simulink model "mcb_pmsm_foc_hall_f28069m_Hall_Sensor_Aceleracion"  (R2022b)
settings: Solver=FixedStepDiscrete  StartTime=0.0  StopTime=8  RelTol=1e-3  EnableMultiTasking=on
InitFcn:
  | mcb_pmsm_foc_hall_f28069m_data;
undefined symbols (not defined in the file): Down, GPTRIP1SEL, GPTRIP2SEL, inverter, PI_params, pmsm, target, Ts, Ts_motor, Ts_simulink, Ts_speed, TZ1, TZ2, Up
libraries: simulink x14, mcbcontrolslib x9, mcbpositiondecoderlib x7, idelinklib_common x6, c2802xlib x5, c280xlib x5, slpidlib x3, c2806xlib x3, svdutilitieslib x2, c2000lib x1, mcbplantlib x1, autolibpmsmexterior x1
(part 2 of 3)

== system mcb_pmsm_foc_hall_f28069m_Hall_Sensor_Aceleracion/Hall Sensor C/Capture Event Selection ==
  Hall State : Inport
  If : If  IfExpression=(u1 == 5 | u1 == 6)
  Merge : Merge
  Output 0 : Subsystem  TreatAsAtomicUnit=on
  Output 1 : Subsystem  TreatAsAtomicUnit=on
  Capture Event Select : Outport
  wires:
  Output 1/1(Out1) -> Merge/1
  Output 0/1(Out1) -> Merge/2
  If/2 -> Output 0/Action
  If/1 -> Output 1/Action
  Hall State/1 -> If/1
  Merge/1 -> Capture Event Select/1

== system mcb_pmsm_foc_hall_f28069m_Hall_Sensor_Aceleracion/Hall Sensor C/Code generation ==
  eCAP : c280xlib/eCAP  operatingMode=eCAP  selectCAPx=eCAP3  offsetValue=0  counterSynIn=off  enableCounter=off  syncOutput=Disabled  sampleTime=-1  eventPrescaler=0  selectMode=Continuous  enableOneShot=off  stopValue=Capture Event 2  resetEv1Ts=on  ev1Polarity=Rising Edge  resetEv2Ts=on  ev2Polarity=Falling Edge  resetEv3Ts=off  ev3Polarity=Rising Edge  resetEv4Ts=off  ev4Polarity=Rising Edge  tSCntrDataType=uint32  capEvFlag=off  capFlagDataType=uint16  overFlowFlag=off  overFlowFlagDataType=uint16  periodUnit=Seconds  periodSource=Specify via dialog  waveformPeriod=0.001  dutyUnit=Percentages  dutySource=Specify via dialog  dutyCycle=50  outputPolarity=Active High  enableCEVT1Int=on  enableCEVT2Int=on  enableCEVT3Int=off  enableCEVT4Int=off  enableCTROVFInt=on  enablePRDInt=off  enableCMPInt=off
  eCAP_Out : Outport
  wires:
  eCAP/1 -> eCAP_Out/1

== system mcb_pmsm_foc_hall_f28069m_Hall_Sensor_Aceleracion/Hall Sensor C/CodeGen ==
  Bitwise AND : simulink/Logic and Bit Operations/Bitwise Operator  logicop=AND  UseBitMask=on  BitMask=hex2dec('07000000')  BitMaskRealWorld=Stored Integer
  Data Type Conversion : DataTypeConversion  OutDataTypeStr=uint32  ConvertRealWorld=Stored Integer (SI)  SaturateOnIntegerOverflow=off  RndMeth=Floor
  Memory Copy : idelinklib_common/Memory Copy  copyFrom=Specified source code symbol  copyFromAddressSource=Specify via dialog  copyFromAddress=hex2dec('00001000')  copyFromSrcCode=&GpioDataRegs.GPADAT.all  dataTypeFrom=uint32  dataDimensionFrom=1  useOffsetFrom=off  offsetFromSrc=Specify via dialog  offsetFrom=0  strideFrom=1  copyTo=Output port  copyToAddressSource=Specify via dialog  copyToAddress=hex2dec('00002000')  copyToSrcCode=myVariableDst  dataTypeTo=uint32  useOffsetTo=off  offsetToSrc=Specify via dialog  offsetTo=0  strideTo=1  sampleTime=-1  useInitValue=off  initValueSrc=Specify constant value  initValue=1  initValueSrcCode=myInitValueVariable  useAsMask=off  maskOperator=bitwise AND  useTermValue=off  termValue=1  isRealtimeEnabled=off  emitCCBeforeWrite=off  CCBeforeWrite=/* Custom Code Before Write*/  emitCCAfterWrite=off  CCAfterWrite=/* Custom Code After Write*/
  Shift Arithmetic : ArithShift  BitShiftNumber=24
  Out1 : Outport
  wires:
  Data Type Conversion/1 -> Out1/1
  Shift Arithmetic/1 -> Data Type Conversion/1
  Bitwise AND/1 -> Shift Arithmetic/1
  Memory Copy/1 -> Bitwise AND/1

== system mcb_pmsm_foc_hall_f28069m_Hall_Sensor_Aceleracion/Hall Sensor C/Sim ==
  Data Type Conversion : DataTypeConversion  OutDataTypeStr=uint32  ConvertRealWorld=Stored Integer (SI)  SaturateOnIntegerOverflow=off  RndMeth=Floor
  Ground : Ground
  Out1 : Outport
  wires:
  Data Type Conversion/1 -> Out1/1
  Ground/1 -> Data Type Conversion/1

== system mcb_pmsm_foc_hall_f28069m_Hall_Sensor_Aceleracion/Hall Sensor C/Simulation ==
  Ground : Ground
  Ground1 : Ground
  Mux : Mux  Inputs=2
  Out1 : Outport
  wires:
  Ground1/1 -> Mux/2
  Mux/1 -> Out1/1
  Ground/1 -> Mux/1

== system mcb_pmsm_foc_hall_f28069m_Hall_Sensor_Aceleracion/Hardware Init/Code Generation ==
  Input : Inport
  ADC Calib Enable : Constant  Value=inverter.ADCOffsetCalibEnable
  "Calculate ADC Offset " : Subsystem  Priority=1001  TreatAsAtomicUnit=on
  DRV Enable : Subsystem  Priority=1
  Default ADC Offset : Subsystem  Priority=1001  TreatAsAtomicUnit=on
  NOT : Logic  Operator=NOT  IconShape=distinctive  AllPortsSameDT=off  OutDataTypeStr=boolean
  wires:
  Input/1 -> DRV Enable/1(Input)
  ADC Calib Enable/1 -> "Calculate ADC Offset "/Enable, NOT/1
  NOT/1 -> Default ADC Offset/Enable

== system mcb_pmsm_foc_hall_f28069m_Hall_Sensor_Aceleracion/Hardware Init/Simulation ==
  Input : Inport
  Terminator : Terminator
  wires:
  Input/1 -> Terminator/1

== system mcb_pmsm_foc_hall_f28069m_Hall_Sensor_Aceleracion/Heartbeat LED/Code generation ==
  note: Heartbeat LED 1HZ
  In1 : Inport
  Digital Output1 : c2806xlib/Digital Output  GPIO_Number=GPIO24~GPIO31  GPIO_Bit0=off  GPIO_BIT0_Toggle=off  GPIO_Bit1=off  GPIO_BIT1_Toggle=off  GPIO_Bit2=off  GPIO_BIT2_Toggle=off  GPIO_Bit3=off  GPIO_BIT3_Toggle=off  GPIO_Bit4=off  GPIO_BIT4_Toggle=off  GPIO_Bit5=off  GPIO_BIT5_Toggle=off  GPIO_Bit6=off  GPIO_BIT6_Toggle=off  GPIO_Bit7=on  GPIO_BIT7_Toggle=on
  wires:
  In1/1 -> Digital Output1/1

== system mcb_pmsm_foc_hall_f28069m_Hall_Sensor_Aceleracion/Heartbeat LED/Simulation ==
  In1 : Inport
  Simulation_Terminator : Terminator
  wires:
  In1/1 -> Simulation_Terminator/1

== system mcb_pmsm_foc_hall_f28069m_Hall_Sensor_Aceleracion/Inverter and Motor - Plant Model/Codegeneration ==
  Duty_Cycles : Inport
  Ground : Ground
  Ground1 : Ground
  Terminator : Terminator
  Iab_fb_Sim : Outport  VectorParamsAs1DForOutWhenUnconnected=off
  Pos_fb_Sim : Outport  Port=2  VectorParamsAs1DForOutWhenUnconnected=off
  wires:
  Duty_Cycles/1 -> Terminator/1
  Ground/1 -> Iab_fb_Sim/1
  Ground1/1 -> Pos_fb_Sim/1

== system mcb_pmsm_foc_hall_f28069m_Hall_Sensor_Aceleracion/Inverter and Motor - Plant Model/Simulation ==
  Duty_Cycles : Inport
  Inverter : Subsystem
  Load_Profile (Torque) : Subsystem
  RT1 : RateTransition  Deterministic=off  OutPortSampleTime=Ts_simulink
  RT3 : RateTransition  Deterministic=off  OutPortSampleTime=Ts_simulink
  Rate Transition : RateTransition  Deterministic=off  OutPortSampleTime=Ts_motor
  Rate Transition1 : RateTransition  Deterministic=off  OutPortSampleTime=Ts_motor
  Sensor_Measurements : Subsystem
  Surface Mount PMSM : autolibpmsmexterior/Surface Mount PMSM  port_config=Torque  sim_type=Discrete  Ts=Ts_motor  P=pmsm.p  Rs=pmsm.Rs + inverter.R_board  Ldq_=pmsm.Ld  KConstText=Permanent flux linkage constant (lambda_pm):  lambda_pm=pmsm.FluxPM  Ke=159.9771  Kt=1.323  mechanical=[pmsm.J, pmsm.B, 0]  idq0=[0 0]  theta_init=0  omega_init=0  KConst=pmsm.FluxPM  lambda_pm_calc=pmsm.FluxPM  RefBlkName='autolibpmsmexterior/Surface Mount PMSM'  aMode=5  Ldq="[0.0006      0.0006]"
  Terminator : Terminator
  Iab_fb_Sim : Outport  VectorParamsAs1DForOutWhenUnconnected=off
  Pos_fb_Sim : Outport  Port=2  VectorParamsAs1DForOutWhenUnconnected=off
  wires:
  RT1/1 -> Sensor_Measurements/2(PhaseCurr)
  Surface Mount PMSM/3 -> Terminator/1
  Inverter/1(Vabc) -> Rate Transition/1
  Load_Profile (Torque)/1(Load_Trq) -> Rate Transition1/1
  Surface Mount PMSM/2 -> RT1/1  "Iabc"
  RT3/1 -> Sensor_Measurements/1(Info)
  Surface Mount PMSM/1 -> RT3/1
  Rate Transition1/1 -> Surface Mount PMSM/1
  Rate Transition/1 -> Surface Mount PMSM/2
  Duty_Cycles/1 -> Inverter/1(Duty_abc)
  Sensor_Measurements/1(Iab_fb) -> Iab_fb_Sim/1
  Sensor_Measurements/2(Pos_fb) -> Pos_fb_Sim/1

== system mcb_pmsm_foc_hall_f28069m_Hall_Sensor_Aceleracion/Serial Receive/Code Generation ==
  SCI Receive : c280xlib/SCI Receive  sciModule=A  dataHead=''  headerCheckMaxCount=16  dataTail=''  dataType=uint16  dataLenOptions=Length via dialog  dataDim=2  maxDataLength=1  initValue=0  errOption=Output the last received value  errValue=0  sampleTime=-1  blockingMode=on  timeOut=0.019444  outputStatus=off
  Data : Outport
  wires:
  SCI Receive/1 -> Data/1

== system mcb_pmsm_foc_hall_f28069m_Hall_Sensor_Aceleracion/Serial Receive/Data_Conditioning ==
  In1 : Inport
  Data Type Conversion1 : DataTypeConversion  OutDataTypeStr=single  RndMeth=Simplest  SaturateOnIntegerOverflow=off
  Data Type Conversion2 : DataTypeConversion  OutDataTypeStr=fixdt(1,16,12)  ConvertRealWorld=Stored Integer (SI)  RndMeth=Simplest  SaturateOnIntegerOverflow=off
  Out1 : Outport  VectorParamsAs1DForOutWhenUnconnected=off
  wires:
  Data Type Conversion1/1 -> Out1/1
  In1/1 -> Data Type Conversion2/1
  Data Type Conversion2/1 -> Data Type Conversion1/1

== system mcb_pmsm_foc_hall_f28069m_Hall_Sensor_Aceleracion/Serial Receive/Simulation ==
  Data Type Conversion : DataTypeConversion  OutDataTypeStr=fixdt(1,16,12)  RndMeth=Simplest  SaturateOnIntegerOverflow=off
  Data Type Conversion2 : DataTypeConversion  OutDataTypeStr=single  RndMeth=Simplest  SaturateOnIntegerOverflow=off
  Data Type Conversion3 : DataTypeConversion  OutDataTypeStr=uint32  ConvertRealWorld=Stored Integer (SI)  RndMeth=Simplest  SaturateOnIntegerOverflow=off
  Data Type Conversion4 : DataTypeConversion  OutDataTypeStr=single  RndMeth=Simplest  SaturateOnIntegerOverflow=off
  Enable : Constant  OutDataTypeStr=dataType  SampleTime=-1
  Mux : Mux  Inputs=2
  Reversal : Step  Time=6  After=0.1
  Speed_Ref_Final (rpm) : Constant  Value=0.3*pmsm.N_base  OutDataTypeStr=dataType  SampleTime=-1
  Speed_Ref_Init (rpm) : Step  Time=4  Before=0.2*pmsm.N_base  After=0.8*pmsm.N_base
  Switch : Switch  Criteria=u2 > Threshold  SaturateOnIntegerOverflow=off  InputSameDT=off
  rpm2PU : Gain  Gain=1/pmsm.N_base  RndMeth=Simplest  OutDataTypeStr=Inherit: Same as input
  Data : Outport
  wires:
  Data Type Conversion3/1 -> Data/1
  Switch/1 -> rpm2PU/1
  rpm2PU/1 -> Data Type Conversion2/1
  Data Type Conversion4/1 -> Mux/2
  Enable/1 -> Data Type Conversion4/1
  Data Type Conversion2/1 -> Mux/1
  Speed_Ref_Final (rpm)/1 -> Switch/1
  Reversal/1 -> Switch/2
  Speed_Ref_Init (rpm)/1 -> Switch/3
  Data Type Conversion/1 -> Data Type Conversion3/1
  Mux/1 -> Data Type Conversion/1

== system mcb_pmsm_foc_hall_f28069m_Hall_Sensor_Aceleracion/Speed Control/PI_Controller_Speed ==
  N_ref : Inport
  N_fb : Inport  Port=2
  Data Store Read1 : DataStoreRead  DataStoreName=Enable  IndexOptions=Index vector (dialog)  Indices=1  OutputSizes=1
  Discrete PI Controller with anti-windup & reset : slpidlib/PID Controller  Controller=PI  Form=Parallel  TimeDomain=Discrete-time  UseExternalTs=off  SampleTime=-1  IntegratorMethod=Forward Euler  FilterMethod=Forward Euler  ControllerParametersSource=external  P=1  I=1  UseKiTs=on  D=0  N=100  UseFilter=on  TunerSelectOption=Transfer Function Based (PID Tuner App)  InitialConditionSource=external  InitialConditionForIntegrator=0  InitialConditionForFilter=0  DifferentiatorICPrevScaledInput=0  ExternalReset=level  TrackingMode=off  Kt=1  LimitOutput=on  SatLimitsSource=internal  UpperSaturationLimit=1  LowerSaturationLimit=-1  LinearizeAsGain=on  AntiWindupMode=clamping  Kb=1  LimitIntegrator=off  UpperIntegratorSaturationLimit=inf  LowerIntegratorSaturationLimit=-inf  RndMeth=Simplest  POutMin=[]  POutMax=[]  IOutMin=[]  IOutMax=[]  DOutMin=[]  DOutMax=[]  NOutMin=[]  NOutMax=[]  SumOutMin=[]  SumOutMax=[]  SaturationOutDataTypeStr=Inherit: Inherit via back propagation  SaturationOutMin=[]  SaturationOutMax=[]  PParamMin=[]  PParamMax=[]  IParamMin=[]  IParamMax=[]  DParamMin=[]  DParamMax=[]  NParamMin=[]  NParamMax=[]  KbParamMin=[]  KbParamMax=[]  KtParamMin=[]  KtParamMax=[]  KbOutMin=[]  KbOutMax=[]  KtOutMin=[]  KtOutMax=[]  IntegratorOutMin=[]  IntegratorOutMax=[]  FilterOutMin=[]  FilterOutMax=[]  SumI1OutMin=[]  SumI1OutMax=[]  SumI2OutMin=[]  SumI2OutMax=[]  SumI3OutMin=[]  SumI3OutMax=[]  SumI4OutMin=[]  SumI4OutMax=[]  SumDOutMin=[]  SumDOutMax=[]  DifferentiatorOutMin=[]  DifferentiatorOutMax=[]  FilterDiffOutCoefMin=[]  FilterDiffOutCoefMax=[]  ReciprocalOutMin=[]  ReciprocalOutMax=[]  SumDenOutMin=[]  SumDenOutMax=[]  SumNumOutMin=[]  SumNumOutMax=[]  DivideOutMin=[]  DivideOutMax=[]  UdiffTsProdOutMin=[]  UdiffTsProdOutMax=[]  NTsProdOutMin=[]  NTsProdOutMax=[]  UintegralTsProdOutMin=[]  UintegralTsProdOutMax=[]  UngainTsProdOutMin=[]  UngainTsProdOutMax=[]  ClampingZeroOutDataTypeStr=Inherit: Inherit via back propagation  ClampingZeroOutMin=[]  ClampingZeroOutMax=[]  FilterDenConstantOutDataTypeStr=Inherit: Inherit via back propagation  FilterDenConstantOutMin=[]  FilterDenConstantOutMax=[]  PCopyOutDataTypeStr=Inherit: Inherit via back propagation  PCopyOutMin=[]  PCopyOutMax=[]  NCopyOutDataTypeStr=Inherit: Inherit via back propagation  NCopyOutMin=[]  NCopyOutMax=[]  IntegratorContinuousStateAttributes=''  IntegratorStateMustResolveToSignalObject=off  IntegratorRTWStateStorageClass=Auto  FilterContinuousStateAttributes=''  FilterStateMustResolveToSignalObject=off  FilterRTWStateStorageClass=Auto  ParallelPVariant=ExternalParameters  IdealPVariant=Disabled  IVariant=ExternalParameters  DVariant=Disabled  IntegratorVariant=Discrete  SatVariant=Enabled  AWVariant=DiscClampingParallel  PCopyVariant=Disabled  TRVariant=Disabled  FdbkBlocksVariant=Forward  IdealPFdbkVariant=Disabled  SatFdbkVariant=Disabled  DerivativeFilterVariant=Disabled  NVariant=Disabled  NCopyVariant=Disabled_SignalSpec  FilterICVariant=Disabled  IntegratorICVariant=ExternalICs  ExternalResetVariant=ExternalReset  TRSumVariant=Passthrough  SumFdbkVariant=Disabled  SumVariant=Sum_PI  TsampFilterVariant=InternalTs  TsampNgainVariant=Passthrough  TsampIntegralVariant=Passthrough  ExternalSaturationOutDataTypeStr=Inherit: Same as second input
      settings: LibrarySourceBlock=mcbcontrolslib/PI Controller
  Ki1 : Constant  Value=PI_params.Ki_speed*Ts_speed  OutDataTypeStr=dataType  SampleTime=-1
  Ki2 : Constant  Value=0  OutDataTypeStr=dataType  SampleTime=-1
  Kp1 : Constant  Value=PI_params.Kp_speed  OutDataTypeStr=dataType  SampleTime=-1
  Logical Operator : Logic  Operator=NOT  IconShape=distinctive  AllPortsSameDT=off  OutDataTypeStr=boolean
  Sum : Sum  Inputs=|+-  RndMeth=Simplest  OutDataTypeStr=Inherit: Same as first input
  Iq_ref : Outport  VectorParamsAs1DForOutWhenUnconnected=off
  wires:
  Discrete PI Controller with anti-windup & reset/1 -> Iq_ref/1
  Ki1/1 -> Discrete PI Controller with anti-windup & reset/3
  Kp1/1 -> Discrete PI Controller with anti-windup & reset/2
  N_fb/1 -> Sum/2
  Sum/1 -> Discrete PI Controller with anti-windup & reset/1
  Ki2/1 -> Discrete PI Controller with anti-windup & reset/5
  Data Store Read1/1 -> Logical Operator/1
  Logical Operator/1 -> Discrete PI Controller with anti-windup & reset/4
  N_ref/1 -> Sum/1

== system mcb_pmsm_foc_hall_f28069m_Hall_Sensor_Aceleracion/Speed Control/Speed_Ref_Selector ==
  Speed_Ref_In : Inport
  Speed_Ref_Open : Inport  Port=2
  Data Store Read1 : DataStoreRead  DataStoreName=Enable  IndexOptions=Index vector (dialog)  Indices=1  OutputSizes=1
  IIR Filter : mcbcontrolslib/IIR Filter  VariantControl=Low Pass Filter  VariantSelect=Low-pass  Filter_constant=0.01  advancedSettings=off  Ts=50e-6  cutOff_freq=32.1525
  Switch : Switch  Criteria=u2 > Threshold  Threshold=0.5  SaturateOnIntegerOverflow=off  InputSameDT=off
  Speed_Ref_PU : Outport
  wires:
  IIR Filter/1 -> Speed_Ref_PU/1
  Switch/1 -> IIR Filter/1
  Data Store Read1/1 -> Switch/2
  Speed_Ref_Open/1 -> Switch/3
  Speed_Ref_In/1 -> Switch/1

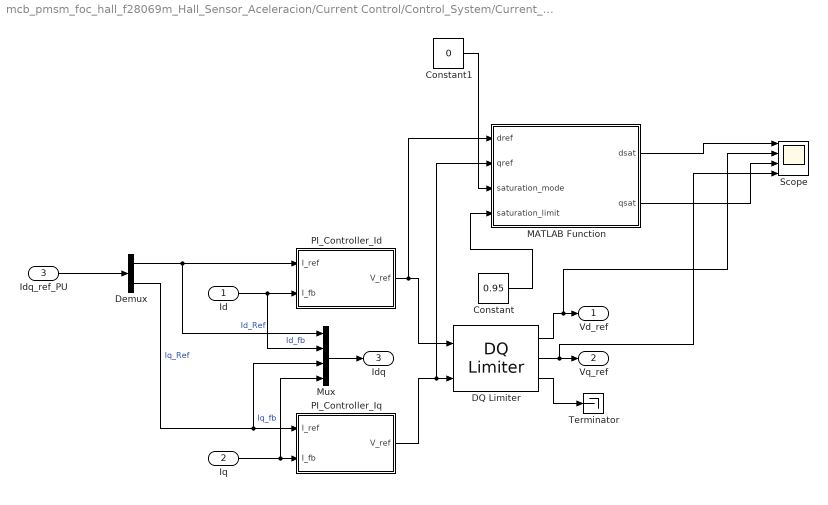
== system mcb_pmsm_foc_hall_f28069m_Hall_Sensor_Aceleracion/Current Control/Control_System/Current_Controllers ==
  Id : Inport
  Iq : Inport  Port=2
  Idq_ref_PU : Inport  Port=3
  Constant : Constant  Value=0.95
  Constant1 : Constant  Value=0
  DQ Limiter : mcbcontrolslib/DQ Limiter  satMethodInputType=Specify via dialog  satMethodSelected=D-Q equivalence  satLimitInputType=Specify via dialog  Vmax=0.95
  Demux : Demux  Outputs=2
  MATLAB Function : MATLAB Function  TreatAsAtomicUnit=on
  Mux : Mux
  PI_Controller_Id : Subsystem
  PI_Controller_Iq : Subsystem
  Scope : Scope  NumInputPorts=4
  Terminator : Terminator
  Vd_ref : Outport  VectorParamsAs1DForOutWhenUnconnected=off
  Vq_ref : Outport  Port=2  VectorParamsAs1DForOutWhenUnconnected=off
  Idq : Outport  Port=3  VectorParamsAs1DForOutWhenUnconnected=off
  wires:
  Iq/1 -> Mux/4, PI_Controller_Iq/2(I_fb)  "Iq_fb"
  Id/1 -> Mux/2, PI_Controller_Id/2(I_fb)  "Id_fb"
  Demux/1 -> Mux/1, PI_Controller_Id/1(I_ref)  "Id_Ref"
  Demux/2 -> Mux/3, PI_Controller_Iq/1(I_ref)  "Iq_Ref"
  PI_Controller_Id/1(V_ref) -> MATLAB Function/1(dref), DQ Limiter/1
  PI_Controller_Iq/1(V_ref) -> MATLAB Function/2(qref), DQ Limiter/2
  Idq_ref_PU/1 -> Demux/1
  DQ Limiter/2 -> Scope/4, Vq_ref/1
  DQ Limiter/1 -> Scope/2, Vd_ref/1
  DQ Limiter/3 -> Terminator/1
  Mux/1 -> Idq/1
  MATLAB Function/1(dsat) -> Scope/1
  MATLAB Function/2(qsat) -> Scope/3
  Constant/1 -> MATLAB Function/4(saturation_limit)
  Constant1/1 -> MATLAB Function/3(saturation_mode)

== system mcb_pmsm_foc_hall_f28069m_Hall_Sensor_Aceleracion/Current Control/Data_Logging/Data ==
  Data : Inport
  Data_width : Inport  Port=2
  Action Port : ActionPort  ActionPortLabel=else
  Mux : Mux  Inputs=2
  Start : Constant  Value=hex2dec('0000')  OutDataTypeStr=uint16
  Data_out : Outport  VectorParamsAs1DForOutWhenUnconnected=off
  Iteration : Outport  Port=2  VectorParamsAs1DForOutWhenUnconnected=off
  wires:
  Start/1 -> Mux/2
  Mux/1 -> Data_out/1
  Data/1 -> Mux/1
  Data_width/1 -> Iteration/1

== system mcb_pmsm_foc_hall_f28069m_Hall_Sensor_Aceleracion/Current Control/Data_Logging/Data_Conditioning ==
  In1 : Inport
  Data Type Conversion : DataTypeConversion  OutDataTypeStr=fixdt(1,32,12)  RndMeth=Simplest  SaturateOnIntegerOverflow=off
  Data Type Conversion3 : DataTypeConversion  OutDataTypeStr=uint16  ConvertRealWorld=Stored Integer (SI)  RndMeth=Simplest  SaturateOnIntegerOverflow=off
  Out1 : Outport  VectorParamsAs1DForOutWhenUnconnected=off
  wires:
  In1/1 -> Data Type Conversion/1
  Data Type Conversion3/1 -> Out1/1
  Data Type Conversion/1 -> Data Type Conversion3/1

== system mcb_pmsm_foc_hall_f28069m_Hall_Sensor_Aceleracion/Current Control/Data_Logging/End ==
  Data : Inport
  Data_width : Inport  Port=2
  Action Port : ActionPort  ActionPortLabel=elseif(u1 == 599)
  Bias : Bias  Bias=1  SaturateOnIntegerOverflow=off
  Mux : Mux  Inputs=2
  Start : Constant  Value=hex2dec('4545')  OutDataTypeStr=uint16
  Data_out : Outport  VectorParamsAs1DForOutWhenUnconnected=off
  Iteration : Outport  Port=2  VectorParamsAs1DForOutWhenUnconnected=off
  wires:
  Mux/1 -> Data_out/1
  Data_width/1 -> Bias/1
  Start/1 -> Mux/2
  Bias/1 -> Iteration/1
  Data/1 -> Mux/1

== system mcb_pmsm_foc_hall_f28069m_Hall_Sensor_Aceleracion/Current Control/Data_Logging/Start ==
  Data : Inport
  Data_width : Inport  Port=2
  Action Port : ActionPort  ActionPortLabel=if(u1 == 0)
  Bias : Bias  Bias=1  SaturateOnIntegerOverflow=off
  End : Constant  Value=hex2dec('5353')  OutDataTypeStr=uint16
  Mux : Mux  Inputs=2
  Data_out : Outport  VectorParamsAs1DForOutWhenUnconnected=off
  Iteration : Outport  Port=2  VectorParamsAs1DForOutWhenUnconnected=off
  wires:
  End/1 -> Mux/1
  Mux/1 -> Data_out/1
  Data_width/1 -> Bias/1
  Bias/1 -> Iteration/1
  Data/1 -> Mux/2

== system mcb_pmsm_foc_hall_f28069m_Hall_Sensor_Aceleracion/Current Control/Input Scaling/Read_Sensor (codegen) ==
  Iab_meas_ADC : Inport  OutDataTypeStr=uint16
  Iab_Sim : Inport  Port=2
  Pos_Sim : Inport  Port=3
  Calculate Position from Hall : Subsystem
  Convert ADC value to PU : Subsystem
  Terminator : Terminator
  Terminator1 : Terminator
  Iab_Meas_PU : Outport  VectorParamsAs1DForOutWhenUnconnected=off
  Pos_PU : Outport  Port=2  VectorParamsAs1DForOutWhenUnconnected=off
  Speed_PU : Outport  Port=3  VectorParamsAs1DForOutWhenUnconnected=off
  wires:
  Iab_Sim/1 -> Terminator/1
  Calculate Position from Hall/1(Pos_PU) -> Pos_PU/1
  Iab_meas_ADC/1 -> Convert ADC value to PU/1(Iab_meas_ADC)
  Convert ADC value to PU/1(Iab_meas_PU) -> Iab_Meas_PU/1
  Pos_Sim/1 -> Terminator1/1
  Calculate Position from Hall/2(Speed_PU) -> Speed_PU/1

== system mcb_pmsm_foc_hall_f28069m_Hall_Sensor_Aceleracion/Current Control/Input Scaling/Read_Sensor (sim) ==
  Iab_meas_ADC : Inport
  Iab_Sim : Inport  Port=2
  Pos_Sim : Inport  Port=3
  Convert ADC value to PU : Subsystem
  Subsystem : Subsystem
  Terminator : Terminator
  Iab_Meas_PU : Outport  VectorParamsAs1DForOutWhenUnconnected=off
  Pos_PU : Outport  Port=2  VectorParamsAs1DForOutWhenUnconnected=off
  Speed_PU : Outport  Port=3  VectorParamsAs1DForOutWhenUnconnected=off
  wires:
  Iab_meas_ADC/1 -> Terminator/1
  Iab_Sim/1 -> Convert ADC value to PU/1(Iab_meas_ADC)
  Convert ADC value to PU/1(Iab_meas_PU) -> Iab_Meas_PU/1
  Pos_Sim/1 -> Subsystem/1(Pos_Sim)
  Subsystem/1(Theta) -> Pos_PU/1
  Subsystem/2(Speed) -> Speed_PU/1

== system mcb_pmsm_foc_hall_f28069m_Hall_Sensor_Aceleracion/Current Control/SCI (Code Generation)/While Iterator Subsystem ==
  Data : Inport
  Iteration : Inport  Port=2
  Add : Sum  Inputs=+-  OutDataTypeStr=Inherit: Same as first input
  Index Vector : MultiPortSwitch  Inputs=1  SaturateOnIntegerOverflow=off  InputSameDT=off
  SCI Transmit : c280xlib/SCI Transmit  sciModule=A  dataHead=''  dataTail=''  blockingMode=on  outputStatus=off
  While Iterator : WhileIterator  MaxIters=-1  WhileBlockType=do-while  ShowIterationPort=on  OutputDataType=int16
  wires:
  While Iterator/1 -> Add/2, Index Vector/1
  Data/1 -> Index Vector/2
  Index Vector/1 -> SCI Transmit/1
  Add/1 -> While Iterator/1
  Iteration/1 -> Add/1

== system mcb_pmsm_foc_hall_f28069m_Hall_Sensor_Aceleracion/Current Control/Sensor Driver Blocks/Sensor Driver Blocks (codegen) ==
  IA/IB Measurement : c2802xlib/ADC  blkParamProc=C2000  ADCModule=1  samplingMode=Simultaneous sample mode  ADCResolution=12-bit (Single-ended input)  useSOC1=SOC0  useSOC2=SOC0_SOC1  SOCAcquisitionWindow=7  SOCTriggerSource=ePWM1_ADCSOCA  SOCInterruptTrigger=No ADCINT  Ts=-1  dType=uint16  postInterrupt=on  interruptSel=ADCINT1  ADCINTContinuous=on  endma=off  chdma=1  conv1=ADCINA0  conv2=ADCINA1 and ADCINB1  conv1_Type4=ADCIN0  conv2_Type4=ADCIN0 and ADCIN1
  Iab_Meas_ADC : Outport
  wires:
  IA/IB Measurement/1 -> Iab_Meas_ADC/1

== system mcb_pmsm_foc_hall_f28069m_Hall_Sensor_Aceleracion/Current Control/Sensor Driver Blocks/Sensor Driver Blocks (sim) ==
  Ground : Ground
  Iab_Meas_ADC : Outport
  wires:
  Ground/1 -> Iab_Meas_ADC/1

== system mcb_pmsm_foc_hall_f28069m_Hall_Sensor_Aceleracion/Hall Sensor A/Capture Event Selection/Output 0 ==
  Action Port : ActionPort  ActionPortLabel=else
  Constant : Constant  Value=0  OutDataTypeStr=boolean
  Out1 : Outport
  wires:
  Constant/1 -> Out1/1

== system mcb_pmsm_foc_hall_f28069m_Hall_Sensor_Aceleracion/Hall Sensor A/Capture Event Selection/Output 1 ==
  Action Port : ActionPort  ActionPortLabel=if((u1 == 5 | u1 == 3))
  Constant : Constant  OutDataTypeStr=boolean
  Out1 : Outport
  wires:
  Constant/1 -> Out1/1

== system mcb_pmsm_foc_hall_f28069m_Hall_Sensor_Aceleracion/Hall Sensor B/Capture Event Selection/Output 0 ==
  Action Port : ActionPort  ActionPortLabel=else
  Constant : Constant  Value=0  OutDataTypeStr=boolean
  Out1 : Outport
  wires:
  Constant/1 -> Out1/1

== system mcb_pmsm_foc_hall_f28069m_Hall_Sensor_Aceleracion/Hall Sensor B/Capture Event Selection/Output 1 ==
  Action Port : ActionPort  ActionPortLabel=if((u1 == 3 | u1 == 6))
  Constant : Constant  OutDataTypeStr=boolean
  Out1 : Outport
  wires:
  Constant/1 -> Out1/1

== system mcb_pmsm_foc_hall_f28069m_Hall_Sensor_Aceleracion/Hall Sensor C/Capture Event Selection/Output 0 ==
  Action Port : ActionPort  ActionPortLabel=else
  Constant : Constant  Value=0  OutDataTypeStr=boolean
  Out1 : Outport
  wires:
  Constant/1 -> Out1/1

== system mcb_pmsm_foc_hall_f28069m_Hall_Sensor_Aceleracion/Hall Sensor C/Capture Event Selection/Output 1 ==
  Action Port : ActionPort  ActionPortLabel=if((u1 == 5 | u1 == 6))
  Constant : Constant  OutDataTypeStr=boolean
  Out1 : Outport
  wires:
  Constant/1 -> Out1/1

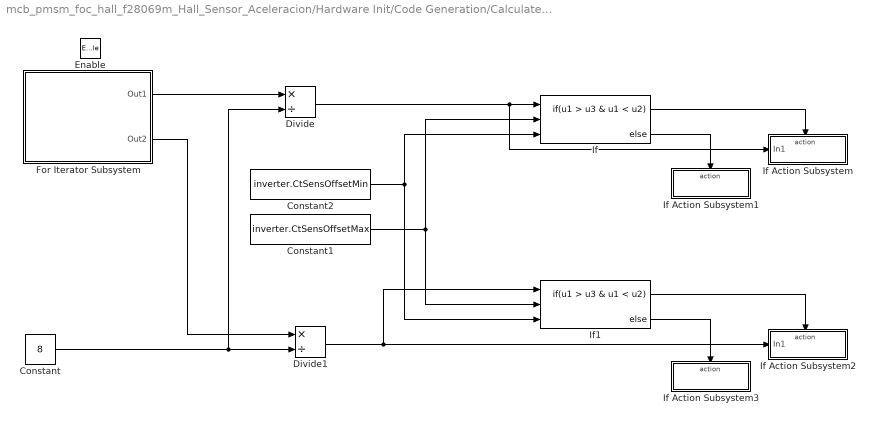
== system mcb_pmsm_foc_hall_f28069m_Hall_Sensor_Aceleracion/Hardware Init/Code Generation/Calculate ADC Offset  ==
  Enable : EnablePort
  Constant : Constant  Value=8
  Constant1 : Constant  Value=inverter.CtSensOffsetMax  OutDataTypeStr=Inherit: Inherit via back propagation
  Constant2 : Constant  Value=inverter.CtSensOffsetMin  OutDataTypeStr=Inherit: Inherit via back propagation
  Divide : Product  Inputs=*/  OutDataTypeStr=uint16
  Divide1 : Product  Inputs=*/  OutDataTypeStr=uint16
  For Iterator Subsystem : Subsystem  TreatAsAtomicUnit=on
  If : If  NumInputs=3  IfExpression=u1 > u3 & u1 < u2
  If Action Subsystem : Subsystem  TreatAsAtomicUnit=on
  If Action Subsystem1 : Subsystem  TreatAsAtomicUnit=on
  If Action Subsystem2 : Subsystem  TreatAsAtomicUnit=on
  If Action Subsystem3 : Subsystem  TreatAsAtomicUnit=on
  If1 : If  NumInputs=3  IfExpression=u1 > u3 & u1 < u2
  wires:
  If1/1 -> If Action Subsystem2/Action
  Constant2/1 -> If/3, If1/3
  Divide1/1 -> If Action Subsystem2/1(In1), If1/1
  If1/2 -> If Action Subsystem3/Action
  If/2 -> If Action Subsystem1/Action
  Constant1/1 -> If1/2, If/2
  If/1 -> If Action Subsystem/Action
  For Iterator Subsystem/1(Out1) -> Divide/1
  For Iterator Subsystem/2(Out2) -> Divide1/1
  Constant/1 -> Divide/2, Divide1/2
  Divide/1 -> If/1, If Action Subsystem/1(In1)

== system mcb_pmsm_foc_hall_f28069m_Hall_Sensor_Aceleracion/Hardware Init/Code Generation/DRV Enable ==
  note: Enable PWM output
  Input : Inport
  Digital Output2 : c2806xlib/Digital Output  GPIO_Number=GPIO0~GPIO7  GPIO_Bit0=off  GPIO_BIT0_Toggle=off  GPIO_Bit1=on  GPIO_BIT1_Toggle=off  GPIO_Bit2=off  GPIO_BIT2_Toggle=off  GPIO_Bit3=on  GPIO_BIT3_Toggle=off  GPIO_Bit4=off  GPIO_BIT4_Toggle=off  GPIO_Bit5=on  GPIO_BIT5_Toggle=off  GPIO_Bit6=off  GPIO_BIT6_Toggle=off  GPIO_Bit7=off  GPIO_BIT7_Toggle=off
  Mux : Mux  Inputs=3
  wires:
  Input/1 -> Mux/3, Mux/1, Mux/2
  Mux/1 -> Digital Output2/1

== system mcb_pmsm_foc_hall_f28069m_Hall_Sensor_Aceleracion/Hardware Init/Code Generation/Default ADC Offset ==
  Enable : EnablePort
  Constant : Constant  Value=inverter.CtSensAOffset  OutDataTypeStr=Inherit: Inherit via back propagation
  Constant1 : Constant  Value=inverter.CtSensBOffset  OutDataTypeStr=Inherit: Inherit via back propagation
  Data Store Write1 : DataStoreWrite  DataStoreName=IaOffset  IndexOptions=Index vector (dialog)  Indices=1  OutputSizes=1
  Data Store Write2 : DataStoreWrite  DataStoreName=IbOffset  IndexOptions=Index vector (dialog)  Indices=1  OutputSizes=1
  wires:
  Constant/1 -> Data Store Write1/1
  Constant1/1 -> Data Store Write2/1

== system mcb_pmsm_foc_hall_f28069m_Hall_Sensor_Aceleracion/Inverter and Motor - Plant Model/Simulation/Inverter ==
  Duty_abc : Inport
  Average-Value Inverter : mcbplantlib/Average-Value Inverter
  Constant2 : Constant  Value=inverter.V_dc  OutDataTypeStr=single  SampleTime=-1
  Data Type Conversion1 : DataTypeConversion  OutDataTypeStr=single  RndMeth=Simplest  SaturateOnIntegerOverflow=off
  Rate Transition3 : RateTransition  Deterministic=off  OutPortSampleTime=Ts_inverter
  Vabc : Outport  VectorParamsAs1DForOutWhenUnconnected=off
  wires:
  Data Type Conversion1/1 -> Rate Transition3/1
  Duty_abc/1 -> Data Type Conversion1/1
  Rate Transition3/1 -> Average-Value Inverter/1
  Constant2/1 -> Average-Value Inverter/2
  Average-Value Inverter/1 -> Vabc/1

== system mcb_pmsm_foc_hall_f28069m_Hall_Sensor_Aceleracion/Inverter and Motor - Plant Model/Simulation/Load_Profile (Torque) ==
  Data Type Conversion : DataTypeConversion  OutDataTypeStr=single  SaturateOnIntegerOverflow=off  RndMeth=Floor
  IIR Filter : mcbcontrolslib/IIR Filter  VariantControl=Low Pass Filter  VariantSelect=Low-pass  Filter_constant=0.01  advancedSettings=off  Ts=50e-6  cutOff_freq=32.1525
  T_load : Step  Time=5  Before=0.05*pmsm.T_rated  After=0.5*pmsm.T_rated  SampleTime=Ts_simulink
  Load_Trq : Outport  VectorParamsAs1DForOutWhenUnconnected=off
  wires:
  T_load/1 -> Data Type Conversion/1
  Data Type Conversion/1 -> IIR Filter/1
  IIR Filter/1 -> Load_Trq/1

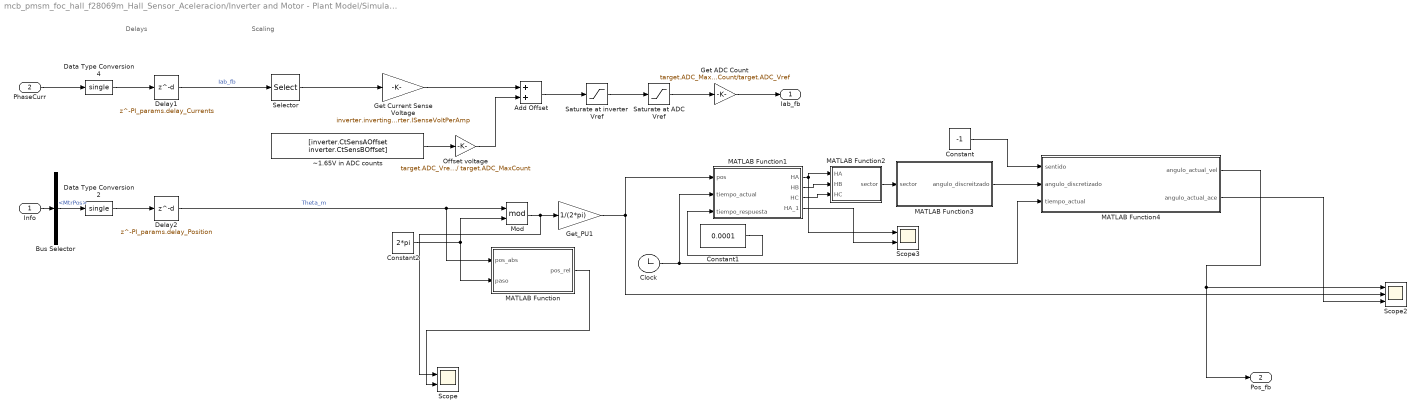
== system mcb_pmsm_foc_hall_f28069m_Hall_Sensor_Aceleracion/Inverter and Motor - Plant Model/Simulation/Sensor_Measurements ==
  note: Scaling
  note: Delays
  Info : Inport
  PhaseCurr : Inport  Port=2
  Add Offset : Sum  RndMeth=Simplest
  Bus Selector : BusSelector  OutputSignals=MtrPos
  Clock : Clock
  Constant : Constant  Value=-1
  Constant1 : Constant  Value=0.0001
  Constant2 : Constant  Value=2*pi  OutDataTypeStr=single  SampleTime=-1
  Data Type Conversion2 : DataTypeConversion  OutDataTypeStr=single  RndMeth=Simplest  SaturateOnIntegerOverflow=off
  Data Type Conversion4 : DataTypeConversion  OutDataTypeStr=single  RndMeth=Simplest  SaturateOnIntegerOverflow=off
  Delay1 : Delay  DelayLength=PI_params.delay_Currents
  Delay2 : Delay  DelayLength=PI_params.delay_Position
  Get ADC Count : Gain  Gain=target.ADC_MaxCount/target.ADC_Vref  OutMin=0  OutMax=target.ADC_MaxCount  OutDataTypeStr=uint16  RndMeth=Simplest
  Get Current Sense Voltage : Gain  Gain=inverter.invertingAmp * inverter.ISenseVoltPerAmp  RndMeth=Simplest  OutDataTypeStr=Inherit: Same as input
  Get_PU1 : Gain  Gain=1/(2*pi)  OutDataTypeStr=dataType  RndMeth=Simplest
  MATLAB Function : MATLAB Function  TreatAsAtomicUnit=on
  MATLAB Function1 : MATLAB Function  TreatAsAtomicUnit=on
  MATLAB Function2 : MATLAB Function  TreatAsAtomicUnit=on
  MATLAB Function3 : MATLAB Function  TreatAsAtomicUnit=on
  MATLAB Function4 : MATLAB Function  TreatAsAtomicUnit=on
  Mod : Math  Operator=mod
  Offset voltage : Gain  Gain=target.ADC_Vref / target.ADC_MaxCount  RndMeth=Simplest
  Saturate at ADC Vref : Saturate  UpperLimit=target.ADC_Vref  LowerLimit=0
  Saturate at inverter Vref : Saturate  UpperLimit=inverter.ISenseVref  LowerLimit=0
  Scope : Scope  NumInputPorts=2
  Scope2 : Scope  NumInputPorts=3
  Scope3 : Scope  NumInputPorts=2
  Selector : Selector  InputPortWidth=3  IndexOptions=Index vector (dialog)  Indices=[1 2]  OutputSizes=1
  ~1.65V in ADC counts : Constant  Value=[inverter.CtSensAOffset inverter.CtSensBOffset]  OutDataTypeStr=uint16  SampleTime=-1
  Iab_fb : Outport  VectorParamsAs1DForOutWhenUnconnected=off
  Pos_fb : Outport  Port=2  VectorParamsAs1DForOutWhenUnconnected=off
  wires:
  Delay1/1 -> Selector/1  "Iab_fb"
  Data Type Conversion4/1 -> Delay1/1
  PhaseCurr/1 -> Data Type Conversion4/1
  Info/1 -> Bus Selector/1
  Bus Selector/1 -> Data Type Conversion2/1  "<MtrPos>"
  Data Type Conversion2/1 -> Delay2/1
  Delay2/1 -> MATLAB Function/1(pos_abs), Mod/1  "Theta_m"
  Get_PU1/1 -> MATLAB Function1/1(pos), Scope2/2
  Mod/1 -> Scope/1, Get_PU1/1
  Constant2/1 -> MATLAB Function/2(paso), Mod/2
  Get ADC Count/1 -> Iab_fb/1
  Selector/1 -> Get Current Sense Voltage/1
  Add Offset/1 -> Saturate at inverter Vref/1
  Get Current Sense Voltage/1 -> Add Offset/1
  ~1.65V in ADC counts/1 -> Offset voltage/1
  Saturate at inverter Vref/1 -> Saturate at ADC Vref/1
  Offset voltage/1 -> Add Offset/2
  Saturate at ADC Vref/1 -> Get ADC Count/1
  MATLAB Function/1(pos_rel) -> Scope/2
  MATLAB Function1/1(HA) -> Scope3/1, MATLAB Function2/1(HA)
  MATLAB Function1/2(HB) -> MATLAB Function2/2(HB)
  MATLAB Function1/3(HC) -> MATLAB Function2/3(HC)
  MATLAB Function2/1(sector) -> MATLAB Function3/1(sector)
  Clock/1 -> MATLAB Function1/2(tiempo_actual), MATLAB Function4/3(tiempo_actual)
  MATLAB Function3/1(angulo_discreitzado) -> MATLAB Function4/2(angulo_discretizado)
  Constant/1 -> MATLAB Function4/1(sentido)
  MATLAB Function4/1(angulo_actual_vel) -> Pos_fb/1, Scope2/1
  Constant1/1 -> MATLAB Function1/3(tiempo_respuesta)
  MATLAB Function1/4(HA_1) -> Scope3/2
  MATLAB Function4/2(angulo_actual_ace) -> Scope2/3

== system mcb_pmsm_foc_hall_f28069m_Hall_Sensor_Aceleracion/Current Control/Control_System/Current_Controllers/PI_Controller_Id ==
  I_ref : Inport
  I_fb : Inport  Port=2
  Data Store Read1 : DataStoreRead  DataStoreName=Enable  IndexOptions=Index vector (dialog)  Indices=1  OutputSizes=1
  Discrete PI Controller with anti-windup & reset : slpidlib/PID Controller  Controller=PI  Form=Parallel  TimeDomain=Discrete-time  UseExternalTs=off  SampleTime=-1  IntegratorMethod=Forward Euler  FilterMethod=Forward Euler  ControllerParametersSource=external  P=1  I=1  UseKiTs=on  D=0  N=100  UseFilter=on  TunerSelectOption=Transfer Function Based (PID Tuner App)  InitialConditionSource=external  InitialConditionForIntegrator=0  InitialConditionForFilter=0  DifferentiatorICPrevScaledInput=0  ExternalReset=level  TrackingMode=off  Kt=1  LimitOutput=on  SatLimitsSource=internal  UpperSaturationLimit=1  LowerSaturationLimit=-1  LinearizeAsGain=on  AntiWindupMode=clamping  Kb=1  LimitIntegrator=off  UpperIntegratorSaturationLimit=inf  LowerIntegratorSaturationLimit=-inf  RndMeth=Simplest  POutMin=[]  POutMax=[]  IOutMin=[]  IOutMax=[]  DOutMin=[]  DOutMax=[]  NOutMin=[]  NOutMax=[]  SumOutMin=[]  SumOutMax=[]  SaturationOutDataTypeStr=Inherit: Inherit via back propagation  SaturationOutMin=[]  SaturationOutMax=[]  PParamMin=[]  PParamMax=[]  IParamMin=[]  IParamMax=[]  DParamMin=[]  DParamMax=[]  NParamMin=[]  NParamMax=[]  KbParamMin=[]  KbParamMax=[]  KtParamMin=[]  KtParamMax=[]  KbOutMin=[]  KbOutMax=[]  KtOutMin=[]  KtOutMax=[]  IntegratorOutMin=[]  IntegratorOutMax=[]  FilterOutMin=[]  FilterOutMax=[]  SumI1OutMin=[]  SumI1OutMax=[]  SumI2OutMin=[]  SumI2OutMax=[]  SumI3OutMin=[]  SumI3OutMax=[]  SumI4OutMin=[]  SumI4OutMax=[]  SumDOutMin=[]  SumDOutMax=[]  DifferentiatorOutMin=[]  DifferentiatorOutMax=[]  FilterDiffOutCoefMin=[]  FilterDiffOutCoefMax=[]  ReciprocalOutMin=[]  ReciprocalOutMax=[]  SumDenOutMin=[]  SumDenOutMax=[]  SumNumOutMin=[]  SumNumOutMax=[]  DivideOutMin=[]  DivideOutMax=[]  UdiffTsProdOutMin=[]  UdiffTsProdOutMax=[]  NTsProdOutMin=[]  NTsProdOutMax=[]  UintegralTsProdOutMin=[]  UintegralTsProdOutMax=[]  UngainTsProdOutMin=[]  UngainTsProdOutMax=[]  ClampingZeroOutDataTypeStr=Inherit: Inherit via back propagation  ClampingZeroOutMin=[]  ClampingZeroOutMax=[]  FilterDenConstantOutDataTypeStr=Inherit: Inherit via back propagation  FilterDenConstantOutMin=[]  FilterDenConstantOutMax=[]  PCopyOutDataTypeStr=Inherit: Inherit via back propagation  PCopyOutMin=[]  PCopyOutMax=[]  NCopyOutDataTypeStr=Inherit: Inherit via back propagation  NCopyOutMin=[]  NCopyOutMax=[]  IntegratorContinuousStateAttributes=''  IntegratorStateMustResolveToSignalObject=off  IntegratorRTWStateStorageClass=Auto  FilterContinuousStateAttributes=''  FilterStateMustResolveToSignalObject=off  FilterRTWStateStorageClass=Auto  ParallelPVariant=ExternalParameters  IdealPVariant=Disabled  IVariant=ExternalParameters  DVariant=Disabled  IntegratorVariant=Discrete  SatVariant=Enabled  AWVariant=DiscClampingParallel  PCopyVariant=Disabled  TRVariant=Disabled  FdbkBlocksVariant=Forward  IdealPFdbkVariant=Disabled  SatFdbkVariant=Disabled  DerivativeFilterVariant=Disabled  NVariant=Disabled  NCopyVariant=Disabled_SignalSpec  FilterICVariant=Disabled  IntegratorICVariant=ExternalICs  ExternalResetVariant=ExternalReset  TRSumVariant=Passthrough  SumFdbkVariant=Disabled  SumVariant=Sum_PI  TsampFilterVariant=InternalTs  TsampNgainVariant=Passthrough  TsampIntegralVariant=Passthrough  ExternalSaturationOutDataTypeStr=Inherit: Same as second input
      settings: LibrarySourceBlock=mcbcontrolslib/PI Controller
  Ki : Constant  Value=PI_params.Ki_i*Ts  OutDataTypeStr=dataType  SampleTime=-1
  Ki1 : Constant  Value=0  OutDataTypeStr=dataType  SampleTime=-1
  Kp : Constant  Value=PI_params.Kp_i  OutDataTypeStr=dataType  SampleTime=-1
  Logical Operator : Logic  Operator=NOT  IconShape=distinctive  AllPortsSameDT=off  OutDataTypeStr=boolean
  Sum : Sum  Inputs=|+-  OutDataTypeStr=Inherit: Same as first input
  V_ref : Outport  VectorParamsAs1DForOutWhenUnconnected=off
  wires:
  I_ref/1 -> Sum/1
  I_fb/1 -> Sum/2
  Data Store Read1/1 -> Logical Operator/1
  Discrete PI Controller with anti-windup & reset/1 -> V_ref/1
  Sum/1 -> Discrete PI Controller with anti-windup & reset/1
  Kp/1 -> Discrete PI Controller with anti-windup & reset/2
  Ki/1 -> Discrete PI Controller with anti-windup & reset/3
  Logical Operator/1 -> Discrete PI Controller with anti-windup & reset/4
  Ki1/1 -> Discrete PI Controller with anti-windup & reset/5

== system mcb_pmsm_foc_hall_f28069m_Hall_Sensor_Aceleracion/Current Control/Control_System/Current_Controllers/PI_Controller_Iq ==
  I_ref : Inport
  I_fb : Inport  Port=2
  Data Store Read1 : DataStoreRead  DataStoreName=Enable  IndexOptions=Index vector (dialog)  Indices=1  OutputSizes=1
  Discrete PI Controller with anti-windup & reset : slpidlib/PID Controller  Controller=PI  Form=Parallel  TimeDomain=Discrete-time  UseExternalTs=off  SampleTime=-1  IntegratorMethod=Forward Euler  FilterMethod=Forward Euler  ControllerParametersSource=external  P=1  I=1  UseKiTs=on  D=0  N=100  UseFilter=on  TunerSelectOption=Transfer Function Based (PID Tuner App)  InitialConditionSource=external  InitialConditionForIntegrator=0  InitialConditionForFilter=0  DifferentiatorICPrevScaledInput=0  ExternalReset=level  TrackingMode=off  Kt=1  LimitOutput=on  SatLimitsSource=internal  UpperSaturationLimit=1  LowerSaturationLimit=-1  LinearizeAsGain=on  AntiWindupMode=clamping  Kb=1  LimitIntegrator=off  UpperIntegratorSaturationLimit=inf  LowerIntegratorSaturationLimit=-inf  RndMeth=Simplest  POutMin=[]  POutMax=[]  IOutMin=[]  IOutMax=[]  DOutMin=[]  DOutMax=[]  NOutMin=[]  NOutMax=[]  SumOutMin=[]  SumOutMax=[]  SaturationOutDataTypeStr=Inherit: Inherit via back propagation  SaturationOutMin=[]  SaturationOutMax=[]  PParamMin=[]  PParamMax=[]  IParamMin=[]  IParamMax=[]  DParamMin=[]  DParamMax=[]  NParamMin=[]  NParamMax=[]  KbParamMin=[]  KbParamMax=[]  KtParamMin=[]  KtParamMax=[]  KbOutMin=[]  KbOutMax=[]  KtOutMin=[]  KtOutMax=[]  IntegratorOutMin=[]  IntegratorOutMax=[]  FilterOutMin=[]  FilterOutMax=[]  SumI1OutMin=[]  SumI1OutMax=[]  SumI2OutMin=[]  SumI2OutMax=[]  SumI3OutMin=[]  SumI3OutMax=[]  SumI4OutMin=[]  SumI4OutMax=[]  SumDOutMin=[]  SumDOutMax=[]  DifferentiatorOutMin=[]  DifferentiatorOutMax=[]  FilterDiffOutCoefMin=[]  FilterDiffOutCoefMax=[]  ReciprocalOutMin=[]  ReciprocalOutMax=[]  SumDenOutMin=[]  SumDenOutMax=[]  SumNumOutMin=[]  SumNumOutMax=[]  DivideOutMin=[]  DivideOutMax=[]  UdiffTsProdOutMin=[]  UdiffTsProdOutMax=[]  NTsProdOutMin=[]  NTsProdOutMax=[]  UintegralTsProdOutMin=[]  UintegralTsProdOutMax=[]  UngainTsProdOutMin=[]  UngainTsProdOutMax=[]  ClampingZeroOutDataTypeStr=Inherit: Inherit via back propagation  ClampingZeroOutMin=[]  ClampingZeroOutMax=[]  FilterDenConstantOutDataTypeStr=Inherit: Inherit via back propagation  FilterDenConstantOutMin=[]  FilterDenConstantOutMax=[]  PCopyOutDataTypeStr=Inherit: Inherit via back propagation  PCopyOutMin=[]  PCopyOutMax=[]  NCopyOutDataTypeStr=Inherit: Inherit via back propagation  NCopyOutMin=[]  NCopyOutMax=[]  IntegratorContinuousStateAttributes=''  IntegratorStateMustResolveToSignalObject=off  IntegratorRTWStateStorageClass=Auto  FilterContinuousStateAttributes=''  FilterStateMustResolveToSignalObject=off  FilterRTWStateStorageClass=Auto  ParallelPVariant=ExternalParameters  IdealPVariant=Disabled  IVariant=ExternalParameters  DVariant=Disabled  IntegratorVariant=Discrete  SatVariant=Enabled  AWVariant=DiscClampingParallel  PCopyVariant=Disabled  TRVariant=Disabled  FdbkBlocksVariant=Forward  IdealPFdbkVariant=Disabled  SatFdbkVariant=Disabled  DerivativeFilterVariant=Disabled  NVariant=Disabled  NCopyVariant=Disabled_SignalSpec  FilterICVariant=Disabled  IntegratorICVariant=ExternalICs  ExternalResetVariant=ExternalReset  TRSumVariant=Passthrough  SumFdbkVariant=Disabled  SumVariant=Sum_PI  TsampFilterVariant=InternalTs  TsampNgainVariant=Passthrough  TsampIntegralVariant=Passthrough  ExternalSaturationOutDataTypeStr=Inherit: Same as second input
      settings: LibrarySourceBlock=mcbcontrolslib/PI Controller
  Ki : Constant  Value=PI_params.Ki_i*Ts  OutDataTypeStr=dataType  SampleTime=-1
  Kp : Constant  Value=PI_params.Kp_i  OutDataTypeStr=dataType  SampleTime=-1
  Kp1 : Constant  Value=0  OutDataTypeStr=dataType  SampleTime=-1
  Logical Operator : Logic  Operator=NOT  IconShape=distinctive  AllPortsSameDT=off  OutDataTypeStr=boolean
  Sum : Sum  Inputs=|+-  OutDataTypeStr=Inherit: Same as first input
  V_ref : Outport  VectorParamsAs1DForOutWhenUnconnected=off
  wires:
  Discrete PI Controller with anti-windup & reset/1 -> V_ref/1
  Data Store Read1/1 -> Logical Operator/1
  I_fb/1 -> Sum/2
  I_ref/1 -> Sum/1
  Kp/1 -> Discrete PI Controller with anti-windup & reset/2
  Sum/1 -> Discrete PI Controller with anti-windup & reset/1
  Ki/1 -> Discrete PI Controller with anti-windup & reset/3
  Logical Operator/1 -> Discrete PI Controller with anti-windup & reset/4
  Kp1/1 -> Discrete PI Controller with anti-windup & reset/5

== system mcb_pmsm_foc_hall_f28069m_Hall_Sensor_Aceleracion/Current Control/Input Scaling/Read_Sensor (codegen)/Calculate Position from Hall ==
  note: Note: The glitch filter rejects lower values of the speed count input, which resutls in motor speed greater than 10 times Base speed
  Atomic Hall Reading : Subsystem  TreatAsAtomicUnit=on
  Data Store Write2 : DataStoreWrite  Priority=2  DataStoreName=HallStateChangeFlag  IndexOptions=Index vector (dialog)  Indices=1  OutputSizes=1
  Glitch Filter : simulink/Logic and Bit Operations/Compare To Constant  relop=>=  const=target.CPU_frequency * 60 / (pmsm.N_base * 10 * 2 * pmsm.p)  OutDataTypeStr=boolean
  Hall Speed and Position : mcbpositiondecoderlib/Hall Speed and Position  blkExecutionType=Speed and position  CounterSize=32 bits  ClkFreq=target.CPU_frequency  BlkSampleTime=Ts  PolePairs=pmsm.p  MinSpeed=20  HallInterruptConfig=Every 180 Degrees  SpeedUnit=Per unit  PerUnitSpeed=PU_System.N_base  SpeedDataType=dataType  hallSequence=ABC  Sequence=[5,4,6,2,3,1]  EnableSecondOrder=1st Order  PositionUnit=Per unit  PositionDataType=dataType
  Mechanical to Electrical Position : mcbpositiondecoderlib/Mechanical to Electrical Position  NrPP=1  selectedRange=Per unit  MechOfstInputType=Specify via dialog  mechOffsetIn=pmsm.PositionOffset  maxAngleIn=1  InputDataType=dataType  VariantSelect=floating-point
  Subsystem : Subsystem
  Pos_PU : Outport  InitialOutput=0  VectorParamsAs1DForOutWhenUnconnected=off
  Speed_PU : Outport  Port=2  InitialOutput=0  VectorParamsAs1DForOutWhenUnconnected=off
  wires:
  Hall Speed and Position/3 -> Data Store Write2/1
  Hall Speed and Position/1 -> Mechanical to Electrical Position/1
  Mechanical to Electrical Position/1 -> Pos_PU/1
  Hall Speed and Position/2 -> Speed_PU/1
  Atomic Hall Reading/1(HallState) -> Hall Speed and Position/1
  Atomic Hall Reading/2(Count) -> Hall Speed and Position/2
  Atomic Hall Reading/4(Dir) -> Hall Speed and Position/4
  Atomic Hall Reading/5(SpeedValidity) -> Hall Speed and Position/5
  Atomic Hall Reading/6(Hallchange) -> Hall Speed and Position/6
  Glitch Filter/1 -> Subsystem/Enable
  Atomic Hall Reading/3(SpeedCount) -> Glitch Filter/1, Subsystem/1(Input)
  Subsystem/1(Output) -> Hall Speed and Position/3

== system mcb_pmsm_foc_hall_f28069m_Hall_Sensor_Aceleracion/Current Control/Input Scaling/Read_Sensor (codegen)/Convert ADC value to PU ==
  Iab_meas_ADC : Inport
  Add : Sum  Inputs=-+
  DRV_8312 EVM is using an inverted amplifier circuit for current sensing : UnaryMinus
  Data Store Read : DataStoreRead  DataStoreName=IaOffset  IndexOptions=Index vector (dialog)  Indices=1  OutputSizes=1
  Data Store Read1 : DataStoreRead  DataStoreName=IbOffset  IndexOptions=Index vector (dialog)  Indices=1  OutputSizes=1
  Data Type Conversion : DataTypeConversion  OutDataTypeStr=int32  ConvertRealWorld=Stored Integer (SI)  SaturateOnIntegerOverflow=off  RndMeth=Floor
  Data Type Conversion1 : DataTypeConversion  OutDataTypeStr=dataType  SaturateOnIntegerOverflow=off  RndMeth=Floor
  Data Type Conversion3 : DataTypeConversion  OutDataTypeStr=fixdt(1,32,17)  ConvertRealWorld=Stored Integer (SI)  RndMeth=Simplest  SaturateOnIntegerOverflow=off
  Mux : Mux  Inputs=2
  Q17 per unit conversion : ArithShift  BitShiftNumber=-6
  Iab_meas_PU : Outport  InitialOutput=0  VectorParamsAs1DForOutWhenUnconnected=off
  wires:
  DRV_8312 EVM is using an inverted amplifier circuit for current sensing/1 -> Data Type Conversion1/1
  Add/1 -> Q17 per unit conversion/1
  Data Type Conversion/1 -> Add/2
  Iab_meas_ADC/1 -> Data Type Conversion/1
  Mux/1 -> Add/1
  Q17 per unit conversion/1 -> Data Type Conversion3/1
  Data Type Conversion3/1 -> DRV_8312 EVM is using an inverted amplifier circuit for current sensing/1
  Data Type Conversion1/1 -> Iab_meas_PU/1
  Data Store Read1/1 -> Mux/2
  Data Store Read/1 -> Mux/1

== system mcb_pmsm_foc_hall_f28069m_Hall_Sensor_Aceleracion/Current Control/Input Scaling/Read_Sensor (sim)/Convert ADC value to PU ==
  Iab_meas_ADC : Inport
  0A in ADC counts : Constant  Value=[inverter.CtSensAOffset inverter.CtSensBOffset]  OutDataTypeStr=int32  SampleTime=-1
  Add : Sum  Inputs=-+
  DRV_8312 EVM is using an inverted amplifier circuit for current sensing : UnaryMinus
  Data Type Conversion : DataTypeConversion  OutDataTypeStr=int32  ConvertRealWorld=Stored Integer (SI)  SaturateOnIntegerOverflow=off  RndMeth=Floor
  Data Type Conversion1 : DataTypeConversion  OutDataTypeStr=dataType  SaturateOnIntegerOverflow=off  RndMeth=Floor
  Data Type Conversion3 : DataTypeConversion  OutDataTypeStr=fixdt(1,32,17)  ConvertRealWorld=Stored Integer (SI)  RndMeth=Simplest  SaturateOnIntegerOverflow=off
  Q17 per unit conversion : ArithShift  BitShiftNumber=-6
  Iab_meas_PU : Outport  InitialOutput=0  VectorParamsAs1DForOutWhenUnconnected=off
  wires:
  Data Type Conversion3/1 -> DRV_8312 EVM is using an inverted amplifier circuit for current sensing/1
  Add/1 -> Q17 per unit conversion/1
  Data Type Conversion/1 -> Add/2
  Iab_meas_ADC/1 -> Data Type Conversion/1
  0A in ADC counts/1 -> Add/1
  Q17 per unit conversion/1 -> Data Type Conversion3/1
  DRV_8312 EVM is using an inverted amplifier circuit for current sensing/1 -> Data Type Conversion1/1
  Data Type Conversion1/1 -> Iab_meas_PU/1

== system mcb_pmsm_foc_hall_f28069m_Hall_Sensor_Aceleracion/Current Control/Input Scaling/Read_Sensor (sim)/Subsystem ==
  Pos_Sim : Inport
  IIR Filter : mcbcontrolslib/IIR Filter  VariantControl=Low Pass Filter  VariantSelect=Low-pass  Filter_constant=0.01  advancedSettings=off  Ts=50e-6  cutOff_freq=32.1525
  Mechanical to Electrical Position : mcbpositiondecoderlib/Mechanical to Electrical Position  NrPP=pmsm.p  selectedRange=Per unit  MechOfstInputType=Specify via dialog  mechOffsetIn=0  maxAngleIn=1  InputDataType=dataType  VariantSelect=floating-point
  Speed Measurement : mcbpositiondecoderlib/Speed Measurement  PositionUnit=Per unit  PositionScalingDatatype=uint32  SpeedCalculationMode=Time interval for speed calculation  SampleTimeAsync=Ts  MaximumApplicationSpeed=6000  SpeedResolution=5e-6  DelayLength=10  MaximumMeasurableSpeed=59999  MeasurableSpeedResolution=2.794e-05  SpeedUnit=Per unit based on dialog  PerUnitSpeed=PU_System.N_base  SpeedDataType=dataType
  Theta : Outport
  Speed : Outport  Port=2
  wires:
  Mechanical to Electrical Position/1 -> Theta/1
  IIR Filter/1 -> Speed/1
  Speed Measurement/1 -> IIR Filter/1
  Pos_Sim/1 -> Speed Measurement/1, Mechanical to Electrical Position/1

== system mcb_pmsm_foc_hall_f28069m_Hall_Sensor_Aceleracion/Hardware Init/Code Generation/Calculate ADC Offset /For Iterator Subsystem ==
  Demux : Demux  Outputs=2
  For Iterator : ForIterator  IterationLimit=16  IterationVariableDataType=uint16
  IA/IB Measurement : c2802xlib/ADC  blkParamProc=C2000  ADCModule=1  samplingMode=Simultaneous sample mode  ADCResolution=12-bit (Single-ended input)  useSOC1=SOC0  useSOC2=SOC2_SOC3  SOCAcquisitionWindow=7  SOCTriggerSource=Software  SOCInterruptTrigger=No ADCINT  Ts=-1  dType=uint16  postInterrupt=off  interruptSel=ADCINT1  ADCINTContinuous=on  endma=off  chdma=1  conv1=ADCINA0  conv2=ADCINA1 and ADCINB1  conv1_Type4=ADCIN0  conv2_Type4=ADCIN0 and ADCIN1
  If : If  IfExpression=u1 > 8  ShowElse=off
  If Action Subsystem : Subsystem  TreatAsAtomicUnit=on
  Out1 : Outport
  Out2 : Outport  Port=2
  wires:
  For Iterator/1 -> If/1
  If Action Subsystem/1(Out1) -> Out1/1
  If Action Subsystem/2(Out2) -> Out2/1
  If/1 -> If Action Subsystem/Action
  Demux/1 -> If Action Subsystem/1(In1)
  Demux/2 -> If Action Subsystem/2(In2)
  IA/IB Measurement/1 -> Demux/1

== system mcb_pmsm_foc_hall_f28069m_Hall_Sensor_Aceleracion/Hardware Init/Code Generation/Calculate ADC Offset /If Action Subsystem ==
  In1 : Inport
  Action Port : ActionPort  ActionPortLabel=if(u1 > 1500 & u1 < 2500)
  Data Store Write1 : DataStoreWrite  DataStoreName=IaOffset  IndexOptions=Index vector (dialog)  Indices=1  OutputSizes=1
  wires:
  In1/1 -> Data Store Write1/1

== system mcb_pmsm_foc_hall_f28069m_Hall_Sensor_Aceleracion/Hardware Init/Code Generation/Calculate ADC Offset /If Action Subsystem1 ==
  Action Port : ActionPort  ActionPortLabel=else
  Constant : Constant  Value=inverter.CtSensAOffset  OutDataTypeStr=Inherit: Inherit via back propagation
  Data Store Write1 : DataStoreWrite  DataStoreName=IaOffset  IndexOptions=Index vector (dialog)  Indices=1  OutputSizes=1
  wires:
  Constant/1 -> Data Store Write1/1
